simulink model "crossbar_array"  (R2023b)
settings: Solver=FixedStepAuto  StartTime=0.0  StopTime=1e-6  FixedStep=1e-9  RelTol=1e-3
libraries: fl_lib x22, nesl_utility x4, ee_lib x4
settings Model: Creator=Ryan  LastModifiedBy=shenjiarun
settings SolverCC: AlgebraicLoopSolver=TrustRegion
settings DebuggingCC: UnconnectedInputMsg=warning  UnconnectedOutputMsg=warning  UnconnectedLineMsg=warning
settings ModelReferenceCC: EnableRefExpFcnMdlSchedulingChecks=on
settings SFSimCC: CustomCodeUndefinedFunction=UseInterfaceOnly

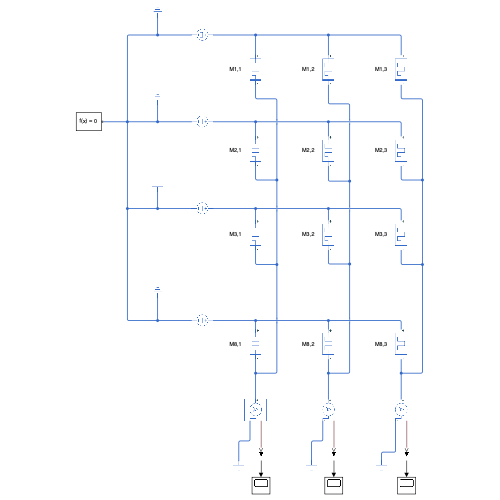
[thumbnail: Simulink's stored preview of the top-level diagram]
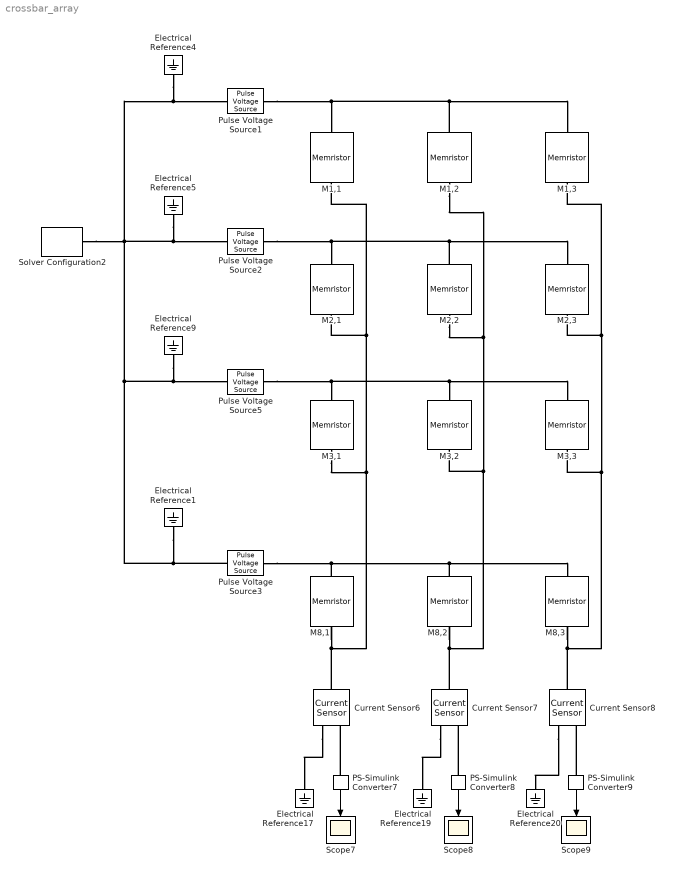
== system crossbar_array ==
  Current Sensor6 : fl_lib/Electrical/Electrical Sensors/Current Sensor
  Current Sensor7 : fl_lib/Electrical/Electrical Sensors/Current Sensor
  Current Sensor8 : fl_lib/Electrical/Electrical Sensors/Current Sensor
  Electrical Reference{1,4..5,9,17,19..20} (7 alike) : fl_lib/Electrical/Electrical Elements/Electrical Reference
  M1,1 : fl_lib/Electrical/Electrical Elements/Memristor  Ra=1 Ohm  Rb=1e2 Ohm  Q0=1e-2 C  x0=0  pwindow=2  i_specify=off  i_priority=None  i=0 A  i_nominal_specify=off  i_nominal_unit=A  i_nominal_value=1  v_specify=off  v_priority=None  v=0 V  v_nominal_specify=off  v_nominal_unit=V  v_nominal_value=1
      settings: InternalSimscapePortConfiguration="{\"Bottom\":[],\"Left\":[{\"id\":\"p\",\"label\":\"+\",\"type\":\"foundation.electrical.electrical\"}],\"Right\":[{\"id\":\"n\",\"label\":\"-\",\"type\":\"foundation.electrical.electrical\"}],\"Top\":[]}"
  M1,2 : fl_lib/Electrical/Electrical Elements/Memristor  Ra=1 Ohm  Rb=1e2 Ohm  Q0=1e-2 C  x0=0  pwindow=2  i_specify=off  i_priority=None  i=0 A  i_nominal_specify=off  i_nominal_unit=A  i_nominal_value=1  v_specify=off  v_priority=None  v=0 V  v_nominal_specify=off  v_nominal_unit=V  v_nominal_value=1
      settings: InternalSimscapePortConfiguration="{\"Bottom\":[],\"Left\":[{\"id\":\"p\",\"label\":\"+\",\"type\":\"foundation.electrical.electrical\"}],\"Right\":[{\"id\":\"n\",\"label\":\"-\",\"type\":\"foundation.electrical.electrical\"}],\"Top\":[]}"
  M1,3 : fl_lib/Electrical/Electrical Elements/Memristor  Ra=1 Ohm  Rb=1e2 Ohm  Q0=1e-2 C  x0=0  pwindow=2  i_specify=off  i_priority=None  i=0 A  i_nominal_specify=off  i_nominal_unit=A  i_nominal_value=1  v_specify=off  v_priority=None  v=0 V  v_nominal_specify=off  v_nominal_unit=V  v_nominal_value=1
      settings: InternalSimscapePortConfiguration="{\"Bottom\":[],\"Left\":[{\"id\":\"p\",\"label\":\"+\",\"type\":\"foundation.electrical.electrical\"}],\"Right\":[{\"id\":\"n\",\"label\":\"-\",\"type\":\"foundation.electrical.electrical\"}],\"Top\":[]}"
  M2,1 : fl_lib/Electrical/Electrical Elements/Memristor  Ra=1 Ohm  Rb=1e2 Ohm  Q0=1e-2 C  x0=0  pwindow=2  i_specify=off  i_priority=None  i=0 A  i_nominal_specify=off  i_nominal_unit=A  i_nominal_value=1  v_specify=off  v_priority=None  v=0 V  v_nominal_specify=off  v_nominal_unit=V  v_nominal_value=1
      settings: InternalSimscapePortConfiguration="{\"Bottom\":[],\"Left\":[{\"id\":\"p\",\"label\":\"+\",\"type\":\"foundation.electrical.electrical\"}],\"Right\":[{\"id\":\"n\",\"label\":\"-\",\"type\":\"foundation.electrical.electrical\"}],\"Top\":[]}"
  M2,2 : fl_lib/Electrical/Electrical Elements/Memristor  Ra=1 Ohm  Rb=1e2 Ohm  Q0=1e-2 C  x0=0  pwindow=2  i_specify=off  i_priority=None  i=0 A  i_nominal_specify=off  i_nominal_unit=A  i_nominal_value=1  v_specify=off  v_priority=None  v=0 V  v_nominal_specify=off  v_nominal_unit=V  v_nominal_value=1
      settings: InternalSimscapePortConfiguration="{\"Bottom\":[],\"Left\":[{\"id\":\"p\",\"label\":\"+\",\"type\":\"foundation.electrical.electrical\"}],\"Right\":[{\"id\":\"n\",\"label\":\"-\",\"type\":\"foundation.electrical.electrical\"}],\"Top\":[]}"
  M2,3 : fl_lib/Electrical/Electrical Elements/Memristor  Ra=1 Ohm  Rb=1e2 Ohm  Q0=1e-2 C  x0=0  pwindow=2  i_specify=off  i_priority=None  i=0 A  i_nominal_specify=off  i_nominal_unit=A  i_nominal_value=1  v_specify=off  v_priority=None  v=0 V  v_nominal_specify=off  v_nominal_unit=V  v_nominal_value=1
      settings: InternalSimscapePortConfiguration="{\"Bottom\":[],\"Left\":[{\"id\":\"p\",\"label\":\"+\",\"type\":\"foundation.electrical.electrical\"}],\"Right\":[{\"id\":\"n\",\"label\":\"-\",\"type\":\"foundation.electrical.electrical\"}],\"Top\":[]}"
  M3,1 : fl_lib/Electrical/Electrical Elements/Memristor  Ra=1 Ohm  Rb=1e2 Ohm  Q0=1e-2 C  x0=0  pwindow=2  i_specify=off  i_priority=None  i=0 A  i_nominal_specify=off  i_nominal_unit=A  i_nominal_value=1  v_specify=off  v_priority=None  v=0 V  v_nominal_specify=off  v_nominal_unit=V  v_nominal_value=1
      settings: InternalSimscapePortConfiguration="{\"Bottom\":[],\"Left\":[{\"id\":\"p\",\"label\":\"+\",\"type\":\"foundation.electrical.electrical\"}],\"Right\":[{\"id\":\"n\",\"label\":\"-\",\"type\":\"foundation.electrical.electrical\"}],\"Top\":[]}"
  M3,2 : fl_lib/Electrical/Electrical Elements/Memristor  Ra=1 Ohm  Rb=1e2 Ohm  Q0=1e-2 C  x0=0  pwindow=2  i_specify=off  i_priority=None  i=0 A  i_nominal_specify=off  i_nominal_unit=A  i_nominal_value=1  v_specify=off  v_priority=None  v=0 V  v_nominal_specify=off  v_nominal_unit=V  v_nominal_value=1
      settings: InternalSimscapePortConfiguration="{\"Bottom\":[],\"Left\":[{\"id\":\"p\",\"label\":\"+\",\"type\":\"foundation.electrical.electrical\"}],\"Right\":[{\"id\":\"n\",\"label\":\"-\",\"type\":\"foundation.electrical.electrical\"}],\"Top\":[]}"
  M3,3 : fl_lib/Electrical/Electrical Elements/Memristor  Ra=1 Ohm  Rb=1e2 Ohm  Q0=1e-2 C  x0=0  pwindow=2  i_specify=off  i_priority=None  i=0 A  i_nominal_specify=off  i_nominal_unit=A  i_nominal_value=1  v_specify=off  v_priority=None  v=0 V  v_nominal_specify=off  v_nominal_unit=V  v_nominal_value=1
      settings: InternalSimscapePortConfiguration="{\"Bottom\":[],\"Left\":[{\"id\":\"p\",\"label\":\"+\",\"type\":\"foundation.electrical.electrical\"}],\"Right\":[{\"id\":\"n\",\"label\":\"-\",\"type\":\"foundation.electrical.electrical\"}],\"Top\":[]}"
  M8,1 : fl_lib/Electrical/Electrical Elements/Memristor  Ra=1 Ohm  Rb=1e2 Ohm  Q0=1e-2 C  x0=0  pwindow=2  i_specify=off  i_priority=None  i=0 A  i_nominal_specify=off  i_nominal_unit=A  i_nominal_value=1  v_specify=off  v_priority=None  v=0 V  v_nominal_specify=off  v_nominal_unit=V  v_nominal_value=1
      settings: InternalSimscapePortConfiguration="{\"Bottom\":[],\"Left\":[{\"id\":\"p\",\"label\":\"+\",\"type\":\"foundation.electrical.electrical\"}],\"Right\":[{\"id\":\"n\",\"label\":\"-\",\"type\":\"foundation.electrical.electrical\"}],\"Top\":[]}"
  M8,2 : fl_lib/Electrical/Electrical Elements/Memristor  Ra=1 Ohm  Rb=1e2 Ohm  Q0=1e-2 C  x0=0  pwindow=2  i_specify=off  i_priority=None  i=0 A  i_nominal_specify=off  i_nominal_unit=A  i_nominal_value=1  v_specify=off  v_priority=None  v=0 V  v_nominal_specify=off  v_nominal_unit=V  v_nominal_value=1
      settings: InternalSimscapePortConfiguration="{\"Bottom\":[],\"Left\":[{\"id\":\"p\",\"label\":\"+\",\"type\":\"foundation.electrical.electrical\"}],\"Right\":[{\"id\":\"n\",\"label\":\"-\",\"type\":\"foundation.electrical.electrical\"}],\"Top\":[]}"
  M8,3 : fl_lib/Electrical/Electrical Elements/Memristor  Ra=1 Ohm  Rb=1e2 Ohm  Q0=1e-2 C  x0=0  pwindow=2  i_specify=off  i_priority=None  i=0 A  i_nominal_specify=off  i_nominal_unit=A  i_nominal_value=1  v_specify=off  v_priority=None  v=0 V  v_nominal_specify=off  v_nominal_unit=V  v_nominal_value=1
      settings: InternalSimscapePortConfiguration="{\"Bottom\":[],\"Left\":[{\"id\":\"p\",\"label\":\"+\",\"type\":\"foundation.electrical.electrical\"}],\"Right\":[{\"id\":\"n\",\"label\":\"-\",\"type\":\"foundation.electrical.electrical\"}],\"Top\":[]}"
  PS-Simulink Converter7 : nesl_utility/PS-Simulink Converter  PhysicalDomain=network_engine_domain  SubClassName=ps_output  LeftPortType=input  RightPortType=output  PseudoPeriodic=off  Frequencies=[]  VectorFormat=1-D array  Unit=1  AffineConversion=off
  PS-Simulink Converter8 : nesl_utility/PS-Simulink Converter  PhysicalDomain=network_engine_domain  SubClassName=ps_output  LeftPortType=input  RightPortType=output  PseudoPeriodic=off  Frequencies=[]  VectorFormat=1-D array  Unit=1  AffineConversion=off
  PS-Simulink Converter9 : nesl_utility/PS-Simulink Converter  PhysicalDomain=network_engine_domain  SubClassName=ps_output  LeftPortType=input  RightPortType=output  PseudoPeriodic=off  Frequencies=[]  VectorFormat=1-D array  Unit=1  AffineConversion=off
  Pulse Voltage Source1 : ee_lib/Additional Components/SPICE Sources/Pulse Voltage Source  V1=0 V  V2=0.15 V  TD=1e-7 s  TR=1e-9 s  TF=1e-9 s  PW=1e-7 s  PER=2e-7 s
      settings: InternalSimscapePortConfiguration="{\"Bottom\":[],\"Left\":[{\"id\":\"p\",\"label\":\"\",\"type\":\"foundation.electrical.electrical\"}],\"Right\":[{\"id\":\"n\",\"label\":\"\",\"type\":\"foundation.electrical.electrical\"}],\"Top\":[]}"
  Pulse Voltage Source2 : ee_lib/Additional Components/SPICE Sources/Pulse Voltage Source  V1=0 V  V2=-0.15 V  TD=1e-7 s  TR=1e-9 s  TF=1e-9 s  PW=1e-7 s  PER=2e-7 s
      settings: InternalSimscapePortConfiguration="{\"Bottom\":[],\"Left\":[{\"id\":\"p\",\"label\":\"\",\"type\":\"foundation.electrical.electrical\"}],\"Right\":[{\"id\":\"n\",\"label\":\"\",\"type\":\"foundation.electrical.electrical\"}],\"Top\":[]}"
  Pulse Voltage Source3 : ee_lib/Additional Components/SPICE Sources/Pulse Voltage Source  V1=0 V  V2=0 V  TD=1e-7 s  TR=1e-9 s  TF=1e-9 s  PW=1e-7 s  PER=2e-7 s
      settings: InternalSimscapePortConfiguration="{\"Bottom\":[],\"Left\":[{\"id\":\"p\",\"label\":\"\",\"type\":\"foundation.electrical.electrical\"}],\"Right\":[{\"id\":\"n\",\"label\":\"\",\"type\":\"foundation.electrical.electrical\"}],\"Top\":[]}"
  Pulse Voltage Source5 : ee_lib/Additional Components/SPICE Sources/Pulse Voltage Source  V1=0 V  V2=0 V  TD=1e-7 s  TR=1e-9 s  TF=1e-9 s  PW=1e-7 s  PER=2e-7 s
      settings: InternalSimscapePortConfiguration="{\"Bottom\":[],\"Left\":[{\"id\":\"p\",\"label\":\"\",\"type\":\"foundation.electrical.electrical\"}],\"Right\":[{\"id\":\"n\",\"label\":\"\",\"type\":\"foundation.electrical.electrical\"}],\"Top\":[]}"
  Scope7 : Scope
  Scope8 : Scope
  Scope9 : Scope
  Solver Configuration2 : nesl_utility/Solver Configuration  PhysicalDomain=network_engine_domain  SubClassName=solver  LeftPortType=input  RightPortType=generic  Tones=[]  Harmonics=[]  SimulateNoise=off  Profile=off  UseLocalSampling=off  EnableSwitchedLinearOptims=on  FrequencyDomain=off  UseCCode=off  RelTol=0.001  AbsTol=1e-06  MinStep=1e-09  ToWorkspace=off  RevertToSquareIcSolve=off  NumHomotopyIterations=100  PhasorMode=off  PhasorModeNumHarmonics=1  ConsistencySolver=NEWTON_FTOL  IndexReductionMethod=DerivativeReplacement  DoDC=off  ResidualTolerance=1e-09  ConsistencyTolSource=GLOBAL  ConsistencyAbsTol=0.001  ConsistencyRelTol=0.001  ConsistencyTolFactor=0.001  UseLocalSolver=off  LocalSolverChoice=NE_BACKWARD_EULER_ADVANCER  ResolveIndetEquations=on  FunctionEvalNumThread=1  LocalSolverSampleTime=0.001  DoFixedCost=off  MaxNonlinIter=3  MaxModeIter=2  ComputeImpulses=off  ImpulseIterations=2  LinearAlgebra=auto  LinearAlgebraNumThread=0  EquationFormulation=NE_TIME_EF  DelaysMemoryBudget=1024  AutomaticFiltering=on  FilteringTimeConstant=0.001  PartitionStorageMethod=AS_NEEDED  PartitionMemoryBudget=1024  PartitionMethod=ROBUST  MultibodyUseLocalSolver=off  MultibodyLocalSolverChoice=ODE1  MultibodyLocalSolverSampleTime=0.001
  wires:
  PS-Simulink Converter7/1 -> Scope7/1
  PS-Simulink Converter8/1 -> Scope8/1
  PS-Simulink Converter9/1 -> Scope9/1
  connections:
  Electrical Reference9/LConn1 -- Electrical Reference1/LConn1 -- Pulse Voltage Source3/RConn1 -- Solver Configuration2/RConn1 -- Pulse Voltage Source2/RConn1 -- Electrical Reference5/LConn1 -- Pulse Voltage Source1/RConn1 -- Electrical Reference4/LConn1 -- Pulse Voltage Source5/RConn1
  Pulse Voltage Source1/LConn1 -- M1,3/LConn1 -- M1,2/LConn1 -- M1,1/LConn1
  M2,3/LConn1 -- M2,2/LConn1 -- M2,1/LConn1 -- Pulse Voltage Source2/LConn1
  M3,3/LConn1 -- M3,2/LConn1 -- M3,1/LConn1 -- Pulse Voltage Source5/LConn1
  M2,1/RConn1 -- M8,1/RConn1 -- Current Sensor6/LConn1 -- M3,1/RConn1 -- M1,1/RConn1
  M2,2/RConn1 -- M1,2/RConn1 -- M8,2/RConn1 -- Current Sensor7/LConn1 -- M3,2/RConn1
  M2,3/RConn1 -- M1,3/RConn1 -- Current Sensor8/LConn1 -- M8,3/RConn1 -- M3,3/RConn1
  PS-Simulink Converter7/LConn1 -- Current Sensor6/RConn1
  PS-Simulink Converter8/LConn1 -- Current Sensor7/RConn1
  PS-Simulink Converter9/LConn1 -- Current Sensor8/RConn1
  Current Sensor6/RConn2 -- Electrical Reference17/LConn1
  Current Sensor7/RConn2 -- Electrical Reference19/LConn1
  Current Sensor8/RConn2 -- Electrical Reference20/LConn1
  Pulse Voltage Source3/LConn1 -- M8,1/LConn1 -- M8,2/LConn1 -- M8,3/LConn1
